simulink model "PIDforVerilog"  (R2024b)
settings: Solver=VariableStepAuto  StartTime=0.0  StopTime=10.0  RelTol=1e-3
undefined symbols (not defined in the file): DiscIntNeverNeededParam
libraries: simulink x6
(part 3 of 3)

== system PIDforVerilog/Discrete PID Controller/Filter/Passthrough ==
  Reset : Inport  SampleTime=SampleTime
  U : Inport  Port=2  SampleTime=SampleTime
  N : Inport  Port=3  SampleTime=SampleTime
  D0in : Inport  Port=4  SampleTime=SampleTime
  Nout : Inport  Port=5  SampleTime=SampleTime
  Ts : Inport  Port=6  SampleTime=SampleTime
  Signal Specification1 : SignalSpecification  DisableCoverage=on  OutDataTypeStr=boolean  SampleTime=SampleTime
  Signal Specification4 : SignalSpecification  DisableCoverage=on  OutDataTypeStr=boolean  SampleTime=SampleTime
  Terminator{1..2,4..6} (5 alike) : Terminator
  Y : Outport  SampleTime=SampleTime
  wires:
  Nout/1 -> Terminator2/1
  Reset/1 -> Terminator5/1
  D0in/1 -> Signal Specification4/1
  Signal Specification4/1 -> Terminator4/1
  N/1 -> Signal Specification1/1
  Signal Specification1/1 -> Terminator1/1
  U/1 -> Y/1
  Ts/1 -> Terminator6/1

== system PIDforVerilog/Discrete PID Controller/Filter ICs/Disabled ==
  D0 : Inport  SampleTime=SampleTime
  Ground : Ground  DisableCoverage=on
  Signal Specification : SignalSpecification  DisableCoverage=on  OutDataTypeStr=boolean  SampleTime=SampleTime
  Signal Specification1 : SignalSpecification  DisableCoverage=on  OutDataTypeStr=boolean  SampleTime=SampleTime
  Terminator : Terminator
  Out1 : Outport  SampleTime=SampleTime
  wires:
  D0/1 -> Signal Specification/1
  Signal Specification/1 -> Terminator/1
  Ground/1 -> Signal Specification1/1
  Signal Specification1/1 -> Out1/1

== system PIDforVerilog/Discrete PID Controller/Filter ICs/External IC ==
  D0 : Inport  SampleTime=SampleTime
  Out1 : Outport  SampleTime=SampleTime
  wires:
  D0/1 -> Out1/1

== system PIDforVerilog/Discrete PID Controller/Filter ICs/Internal IC - Differentiator ==
  D0 : Inport  SampleTime=SampleTime
  Ground : Ground  DisableCoverage=on
  Signal Specification : SignalSpecification  DisableCoverage=on  OutDataTypeStr=boolean  SampleTime=SampleTime
  Signal Specification1 : SignalSpecification  DisableCoverage=on  OutDataTypeStr=boolean  SampleTime=SampleTime
  Terminator : Terminator
  Out1 : Outport  SampleTime=SampleTime
  wires:
  D0/1 -> Signal Specification/1
  Signal Specification/1 -> Terminator/1
  Ground/1 -> Signal Specification1/1
  Signal Specification1/1 -> Out1/1

== system PIDforVerilog/Discrete PID Controller/Filter ICs/Internal IC - Filter ==
  D0 : Inport  OutDataTypeStr=fixdt(1,32,16, 'DataTypeOverride', 'Off')  PortDimensions=1  SampleTime=SampleTime
  Ground : Ground  DisableCoverage=on
  Terminator : Terminator
  Out1 : Outport  OutDataTypeStr=fixdt(1,32,16, 'DataTypeOverride', 'Off')  SampleTime=SampleTime
  wires:
  D0/1 -> Terminator/1
  Ground/1 -> Out1/1

== system PIDforVerilog/Discrete PID Controller/I Gain/Disabled ==
  I Gain : Inport  SampleTime=SampleTime
  Signal Specification : SignalSpecification  DisableCoverage=on  OutDataTypeStr=boolean  SampleTime=SampleTime
  Terminator : Terminator
  wires:
  Signal Specification/1 -> Terminator/1
  I Gain/1 -> Signal Specification/1

== system PIDforVerilog/Discrete PID Controller/I Gain/External Parameters ==
  err : Inport  SampleTime=SampleTime
  I Gain : Inport  Port=2  SampleTime=SampleTime
  IProd Out : Product  OutMin=IOutMin  OutMax=IOutMax  OutDataTypeStr=fixdt(1,32,16, 'DataTypeOverride', 'Off')  SaturateOnIntegerOverflow=on  SampleTime=SampleTime
  Out1 : Outport  SampleTime=SampleTime
  wires:
  err/1 -> IProd Out/1
  I Gain/1 -> IProd Out/2
  IProd Out/1 -> Out1/1

== system PIDforVerilog/Discrete PID Controller/I Gain/Internal Parameters ==
  err : Inport  SampleTime=SampleTime
  I Gain : Inport  Port=2  OutDataTypeStr=fixdt(1,32,16, 'DataTypeOverride', 'Off')  SampleTime=SampleTime
  Integral Gain : Gain  DisableCoverage=on  Gain=I  ParamMin=IParamMin  ParamMax=IParamMax  ParamDataTypeStr=fixdt(1,32,16, 'DataTypeOverride', 'Off')  OutMin=IOutMin  OutMax=IOutMax  OutDataTypeStr=fixdt(1,32,16, 'DataTypeOverride', 'Off')  SaturateOnIntegerOverflow=on
  Terminator : Terminator
  Out1 : Outport  OutDataTypeStr=fixdt(1,32,16, 'DataTypeOverride', 'Off')  SampleTime=SampleTime
  wires:
  err/1 -> Integral Gain/1
  Integral Gain/1 -> Out1/1
  I Gain/1 -> Terminator/1

== system PIDforVerilog/Discrete PID Controller/Ideal P Gain/External Parameters ==
  In1 : Inport  SampleTime=SampleTime
  P Gain : Inport  Port=2  SampleTime=SampleTime
  PProd Out : Product  OutDataTypeStr=fixdt(1,32,16, 'DataTypeOverride', 'Off')  SaturateOnIntegerOverflow=on  SampleTime=SampleTime
  Out1 : Outport  SampleTime=SampleTime
  wires:
  In1/1 -> PProd Out/1
  P Gain/1 -> PProd Out/2
  PProd Out/1 -> Out1/1

== system PIDforVerilog/Discrete PID Controller/Ideal P Gain/Internal Parameters ==
  In1 : Inport  SampleTime=SampleTime
  P Gain : Inport  Port=2  SampleTime=SampleTime
  Proportional Gain : Gain  Gain=P  ParamMin=PParamMin  ParamMax=PParamMax  ParamDataTypeStr=fixdt(1,32,16, 'DataTypeOverride', 'Off')  OutMin=POutMin  OutMax=POutMax  OutDataTypeStr=fixdt(1,32,16, 'DataTypeOverride', 'Off')  SaturateOnIntegerOverflow=on
  Signal Specification1 : SignalSpecification  DisableCoverage=on  OutDataTypeStr=boolean  SampleTime=SampleTime
  Terminator1 : Terminator
  Out1 : Outport  SampleTime=SampleTime
  wires:
  In1/1 -> Proportional Gain/1
  Proportional Gain/1 -> Out1/1
  P Gain/1 -> Signal Specification1/1
  Signal Specification1/1 -> Terminator1/1

== system PIDforVerilog/Discrete PID Controller/Ideal P Gain/Passthrough ==
  In1 : Inport  SampleTime=SampleTime
  P Gain : Inport  Port=2  SampleTime=SampleTime
  Terminator1 : Terminator
  Out1 : Outport  SampleTime=SampleTime
  wires:
  In1/1 -> Out1/1
  P Gain/1 -> Terminator1/1

== system PIDforVerilog/Discrete PID Controller/Ideal P Gain Fdbk/Disabled ==
  In1 : Inport  OutDataTypeStr=fixdt(1,32,16, 'DataTypeOverride', 'Off')  SampleTime=SampleTime
  P Gain : Inport  Port=2  SampleTime=SampleTime
  Terminator1 : Terminator
  Terminator2 : Terminator
  wires:
  P Gain/1 -> Terminator1/1
  In1/1 -> Terminator2/1

== system PIDforVerilog/Discrete PID Controller/Ideal P Gain Fdbk/External Parameters ==
  In1 : Inport  SampleTime=SampleTime
  P Gain : Inport  Port=2  SampleTime=SampleTime
  PProd Out : Product  OutDataTypeStr=fixdt(1,32,16, 'DataTypeOverride', 'Off')  SaturateOnIntegerOverflow=on  SampleTime=SampleTime
  Out1 : Outport  SampleTime=SampleTime
  wires:
  PProd Out/1 -> Out1/1
  P Gain/1 -> PProd Out/2
  In1/1 -> PProd Out/1

== system PIDforVerilog/Discrete PID Controller/Ideal P Gain Fdbk/Internal Parameters ==
  In1 : Inport  SampleTime=SampleTime
  P Gain : Inport  Port=2  SampleTime=SampleTime
  Proportional Gain : Gain  Gain=P  ParamMin=PParamMin  ParamMax=PParamMax  ParamDataTypeStr=fixdt(1,32,16, 'DataTypeOverride', 'Off')  OutMin=POutMin  OutMax=POutMax  OutDataTypeStr=fixdt(1,32,16, 'DataTypeOverride', 'Off')  SaturateOnIntegerOverflow=on
  Signal Specification1 : SignalSpecification  DisableCoverage=on  OutDataTypeStr=boolean  SampleTime=SampleTime
  Terminator1 : Terminator
  Out1 : Outport  SampleTime=SampleTime
  wires:
  Proportional Gain/1 -> Out1/1
  In1/1 -> Proportional Gain/1
  Signal Specification1/1 -> Terminator1/1
  P Gain/1 -> Signal Specification1/1

== system PIDforVerilog/Discrete PID Controller/Ideal P Gain Fdbk/Passthrough ==
  In1 : Inport  SampleTime=SampleTime
  P Gain : Inport  Port=2  SampleTime=SampleTime
  Terminator1 : Terminator
  Out1 : Outport  SampleTime=SampleTime
  wires:
  In1/1 -> Out1/1
  P Gain/1 -> Terminator1/1

== system PIDforVerilog/Discrete PID Controller/Integrator/Continuous ==
  U : Inport  SampleTime=SampleTime
  Reset : Inport  Port=2  SampleTime=SampleTime
  I0in : Inport  Port=3  SampleTime=SampleTime
  Ground : Ground  DisableCoverage=on
  Integrator : Integrator  InitialCondition=InitialConditionForIntegrator  LimitOutput=on  UpperSaturationLimit=UpperIntegratorSaturationLimit  LowerSaturationLimit=LowerIntegratorSaturationLimit  ZeroCross=off
  Signal Specification1 : SignalSpecification  DisableCoverage=on  OutDataTypeStr=boolean  SampleTime=SampleTime
  Terminator : Terminator
  Terminator1 : Terminator
  state : Outport  SampleTime=SampleTime
  out : Outport  Port=2  SampleTime=SampleTime
  wires:
  U/1 -> Integrator/1
  I0in/1 -> Terminator/1
  Integrator/1 -> out/1
  Ground/1 -> Signal Specification1/1
  Signal Specification1/1 -> state/1
  Reset/1 -> Terminator1/1

== system PIDforVerilog/Discrete PID Controller/Integrator/Disabled ==
  U : Inport  SampleTime=SampleTime
  Reset : Inport  Port=2  SampleTime=SampleTime
  I0in : Inport  Port=3  SampleTime=SampleTime
  Ground : Ground  DisableCoverage=on
  Signal Specification1 : SignalSpecification  DisableCoverage=on  OutDataTypeStr=boolean  SampleTime=SampleTime
  Signal Specification2 : SignalSpecification  DisableCoverage=on  OutDataTypeStr=boolean  SampleTime=SampleTime
  Signal Specification4 : SignalSpecification  DisableCoverage=on  OutDataTypeStr=boolean  SampleTime=SampleTime
  Terminator1 : Terminator
  Terminator2 : Terminator
  Terminator3 : Terminator
  out : Outport  SampleTime=SampleTime
  wires:
  Reset/1 -> Terminator2/1
  Signal Specification4/1 -> Terminator1/1
  I0in/1 -> Signal Specification4/1
  U/1 -> Signal Specification1/1
  Signal Specification1/1 -> Terminator3/1
  Ground/1 -> Signal Specification2/1
  Signal Specification2/1 -> out/1

== system PIDforVerilog/Discrete PID Controller/Integrator/Discrete ==
  U : Inport  SampleTime=SampleTime
  Reset : Inport  Port=2  SampleTime=SampleTime
  I0in : Inport  Port=3  SampleTime=SampleTime
  Ground_Integrator : Ground  DisableCoverage=on
  Integrator : DiscreteIntegrator  InitialCondition=InitialConditionForIntegrator  SampleTime=SampleTime  OutMin=IntegratorOutMin  OutMax=IntegratorOutMax  OutDataTypeStr=fixdt(1,32,16, 'DataTypeOverride', 'Off')  SaturateOnIntegerOverflow=on  LimitOutput=on  UpperSaturationLimit=UpperIntegratorSaturationLimit  LowerSaturationLimit=LowerIntegratorSaturationLimit  ICPrevOutput=DiscIntNeverNeededParam  ICPrevScaledInput=DiscIntNeverNeededParam
  Terminator : Terminator
  Terminator1 : Terminator
  Terminator2 : Terminator
  out : Outport  SampleTime=SampleTime
  state : Outport  Port=2  SampleTime=SampleTime
  wires:
  I0in/1 -> Terminator1/1
  Integrator/1 -> out/1
  U/1 -> Integrator/1
  Ground_Integrator/1 -> Terminator/1, state/1
  Reset/1 -> Terminator2/1

== system PIDforVerilog/Discrete PID Controller/Integrator ICs/Disabled ==
  I0 : Inport  SampleTime=SampleTime
  Ground : Ground  DisableCoverage=on
  Signal Specification : SignalSpecification  DisableCoverage=on  OutDataTypeStr=boolean  SampleTime=SampleTime
  Signal Specification1 : SignalSpecification  DisableCoverage=on  OutDataTypeStr=boolean  SampleTime=SampleTime
  Terminator : Terminator
  Out1 : Outport  SampleTime=SampleTime
  wires:
  Signal Specification/1 -> Terminator/1
  I0/1 -> Signal Specification/1
  Signal Specification1/1 -> Out1/1
  Ground/1 -> Signal Specification1/1

== system PIDforVerilog/Discrete PID Controller/Integrator ICs/External IC ==
  I0 : Inport  SampleTime=SampleTime
  Out1 : Outport  SampleTime=SampleTime
  wires:
  I0/1 -> Out1/1

== system PIDforVerilog/Discrete PID Controller/Integrator ICs/Internal IC ==
  I0 : Inport  OutDataTypeStr=fixdt(1,32,16, 'DataTypeOverride', 'Off')  SampleTime=SampleTime
  Ground : Ground  DisableCoverage=on
  Terminator : Terminator
  Out1 : Outport  OutDataTypeStr=fixdt(1,32,16, 'DataTypeOverride', 'Off')  SampleTime=SampleTime
  wires:
  I0/1 -> Terminator/1
  Ground/1 -> Out1/1

== system PIDforVerilog/Discrete PID Controller/N Copy/Disabled ==
  N Gain : Inport  OutDataTypeStr=fixdt(1,32,16, 'DataTypeOverride', 'Off')  SampleTime=SampleTime
  Terminator : Terminator
  wires:
  N Gain/1 -> Terminator/1

== system PIDforVerilog/Discrete PID Controller/N Copy/Disabled wSignal Specification ==
  N Gain : Inport  SampleTime=SampleTime
  Signal Specification1 : SignalSpecification  DisableCoverage=on  OutDataTypeStr=boolean  SampleTime=SampleTime
  Terminator : Terminator
  wires:
  N Gain/1 -> Signal Specification1/1
  Signal Specification1/1 -> Terminator/1

== system PIDforVerilog/Discrete PID Controller/N Copy/External Parameters ==
  N Gain : Inport  SampleTime=SampleTime
  Out1 : Outport  SampleTime=SampleTime
  wires:
  N Gain/1 -> Out1/1

== system PIDforVerilog/Discrete PID Controller/N Copy/Internal Parameters ==
  N Gain : Inport  SampleTime=SampleTime
  N Copy : Constant  DisableCoverage=on  Value=N  OutMin=NCopyOutMin  OutMax=NCopyOutMax  OutDataTypeStr=fixdt(1,32,16, 'DataTypeOverride', 'Off')  PreserveConstantTs=on
  Signal Specification : SignalSpecification  DisableCoverage=on  OutDataTypeStr=boolean  SampleTime=SampleTime
  Terminator : Terminator
  Out1 : Outport  SampleTime=SampleTime
  wires:
  N Copy/1 -> Out1/1
  N Gain/1 -> Signal Specification/1
  Signal Specification/1 -> Terminator/1

== system PIDforVerilog/Discrete PID Controller/N Gain/Disabled ==
  U : Inport  SampleTime=SampleTime
  N Gain : Inport  Port=2  SampleTime=SampleTime
  Signal Specification1 : SignalSpecification  DisableCoverage=on  OutDataTypeStr=boolean  SampleTime=SampleTime
  Signal Specification2 : SignalSpecification  DisableCoverage=on  OutDataTypeStr=boolean  SampleTime=SampleTime
  Terminator1 : Terminator
  Terminator2 : Terminator
  wires:
  Signal Specification2/1 -> Terminator2/1
  U/1 -> Signal Specification2/1
  N Gain/1 -> Signal Specification1/1
  Signal Specification1/1 -> Terminator1/1

== system PIDforVerilog/Discrete PID Controller/N Gain/External Parameters ==
  U : Inport  SampleTime=SampleTime
  N Gain : Inport  Port=2  SampleTime=SampleTime
  NProd Out : Product  OutMin=NOutMin  OutMax=NOutMax  OutDataTypeStr=fixdt(1,32,16, 'DataTypeOverride', 'Off')  SaturateOnIntegerOverflow=on  SampleTime=SampleTime
  Out1 : Outport  SampleTime=SampleTime
  wires:
  U/1 -> NProd Out/1
  N Gain/1 -> NProd Out/2
  NProd Out/1 -> Out1/1

== system PIDforVerilog/Discrete PID Controller/N Gain/Internal Parameters ==
  U : Inport  SampleTime=SampleTime
  N Gain : Inport  Port=2  SampleTime=SampleTime
  Filter Coefficient : Gain  Gain=N  ParamMin=NParamMin  ParamMax=NParamMax  ParamDataTypeStr=fixdt(1,32,16, 'DataTypeOverride', 'Off')  OutMin=NOutMin  OutMax=NOutMax  OutDataTypeStr=fixdt(1,32,16, 'DataTypeOverride', 'Off')  SaturateOnIntegerOverflow=on
  Terminator1 : Terminator
  Out1 : Outport  SampleTime=SampleTime
  wires:
  U/1 -> Filter Coefficient/1
  Filter Coefficient/1 -> Out1/1
  N Gain/1 -> Terminator1/1

== system PIDforVerilog/Discrete PID Controller/N Gain/Passthrough ==
  U : Inport  SampleTime=SampleTime
  N Gain : Inport  Port=2  SampleTime=SampleTime
  Terminator1 : Terminator
  Out1 : Outport  SampleTime=SampleTime
  wires:
  U/1 -> Out1/1
  N Gain/1 -> Terminator1/1

== system PIDforVerilog/Discrete PID Controller/P Copy/Disabled ==
  P Gain : Inport  SampleTime=SampleTime
  Terminator3 : Terminator
  wires:
  P Gain/1 -> Terminator3/1

== system PIDforVerilog/Discrete PID Controller/P Copy/External Parameters Ideal ==
  P Gain : Inport  SampleTime=SampleTime
  Out1 : Outport  SampleTime=SampleTime
  wires:
  P Gain/1 -> Out1/1

== system PIDforVerilog/Discrete PID Controller/P Copy/Internal Parameters Ideal ==
  P Gain : Inport  SampleTime=SampleTime
  P Copy : Constant  DisableCoverage=on  Value=P  OutMin=PCopyOutMin  OutMax=PCopyOutMax  OutDataTypeStr=Inherit: Inherit via back propagation  PreserveConstantTs=on
  Terminator3 : Terminator
  Out1 : Outport  SampleTime=SampleTime
  wires:
  P Copy/1 -> Out1/1
  P Gain/1 -> Terminator3/1

== system PIDforVerilog/Discrete PID Controller/Parallel P Gain/Disabled ==
  P Gain : Inport  SampleTime=SampleTime
  Signal Specification : SignalSpecification  DisableCoverage=on  OutDataTypeStr=boolean  SampleTime=SampleTime
  Terminator : Terminator
  wires:
  P Gain/1 -> Signal Specification/1
  Signal Specification/1 -> Terminator/1

== system PIDforVerilog/Discrete PID Controller/Parallel P Gain/External Parameters ==
  err : Inport  SampleTime=SampleTime
  P Gain : Inport  Port=2  SampleTime=SampleTime
  PProd Out : Product  OutMin=POutMin  OutMax=POutMax  OutDataTypeStr=fixdt(1,32,16, 'DataTypeOverride', 'Off')  SaturateOnIntegerOverflow=on  SampleTime=SampleTime
  Out1 : Outport  SampleTime=SampleTime
  wires:
  PProd Out/1 -> Out1/1
  P Gain/1 -> PProd Out/2
  err/1 -> PProd Out/1

== system PIDforVerilog/Discrete PID Controller/Parallel P Gain/Internal Parameters ==
  err : Inport  SampleTime=SampleTime
  P Gain : Inport  Port=2  OutDataTypeStr=fixdt(1,32,16, 'DataTypeOverride', 'Off')  SampleTime=SampleTime
  Proportional Gain : Gain  Gain=P  ParamMin=PParamMin  ParamMax=PParamMax  ParamDataTypeStr=fixdt(1,32,16, 'DataTypeOverride', 'Off')  OutMin=POutMin  OutMax=POutMax  OutDataTypeStr=fixdt(1,32,16, 'DataTypeOverride', 'Off')  SaturateOnIntegerOverflow=on
  Terminator : Terminator
  Out1 : Outport  SampleTime=SampleTime
  wires:
  Proportional Gain/1 -> Out1/1
  err/1 -> Proportional Gain/1
  P Gain/1 -> Terminator/1

== system PIDforVerilog/Discrete PID Controller/Parallel P Gain/Passthrough ==
  err : Inport  SampleTime=SampleTime
  P Gain : Inport  Port=2  SampleTime=SampleTime
  Terminator : Terminator
  Out1 : Outport  SampleTime=SampleTime
  wires:
  err/1 -> Out1/1
  P Gain/1 -> Terminator/1

== system PIDforVerilog/Discrete PID Controller/Reset Signal/Disabled ==
  Reset : Inport  OutDataTypeStr=fixdt(1,32,16, 'DataTypeOverride', 'Off')  SampleTime=SampleTime
  Ground : Ground  DisableCoverage=on
  Terminator : Terminator
  Out1 : Outport  OutDataTypeStr=fixdt(1,32,16, 'DataTypeOverride', 'Off')  SampleTime=SampleTime
  wires:
  Reset/1 -> Terminator/1
  Ground/1 -> Out1/1

== system PIDforVerilog/Discrete PID Controller/Reset Signal/External Reset ==
  Reset : Inport  SampleTime=SampleTime
  Out1 : Outport  SampleTime=SampleTime
  wires:
  Reset/1 -> Out1/1

== system PIDforVerilog/Discrete PID Controller/Saturation/Enabled ==
  In1 : Inport  SampleTime=SampleTime
  Upper Limit : Inport  Port=2  OutDataTypeStr=fixdt(1,32,16, 'DataTypeOverride', 'Off')  SampleTime=SampleTime
  Lower Limit : Inport  Port=3  OutDataTypeStr=fixdt(1,32,16, 'DataTypeOverride', 'Off')  SampleTime=SampleTime
  Saturation : Saturate  UpperLimit=UpperSaturationLimit  LowerLimit=LowerSaturationLimit  ZeroCross=off  SampleTime=SampleTime  OutMin=SaturationOutMin  OutMax=SaturationOutMax  OutDataTypeStr=fixdt(1,32,16, 'DataTypeOverride', 'Off')
  Terminator : Terminator
  Terminator1 : Terminator
  Out1 : Outport  SampleTime=SampleTime
  wires:
  Lower Limit/1 -> Terminator1/1
  Upper Limit/1 -> Terminator/1
  In1/1 -> Saturation/1
  Saturation/1 -> Out1/1

== system PIDforVerilog/Discrete PID Controller/Saturation/External ==
  In1 : Inport  SampleTime=SampleTime
  Upper Limit : Inport  Port=2  SampleTime=SampleTime
  Lower Limit : Inport  Port=3  SampleTime=SampleTime
  Saturation Dynamic : simulink/Discontinuities/Saturation Dynamic  OutMin=SaturationOutMin  OutMax=SaturationOutMax  OutDataTypeStr=Inherit: Same as second input  OutDataType=fixdt(1, 16)  OutScaling=2^-10  DoSatur=on
  Out1 : Outport  SampleTime=SampleTime
  wires:
  Lower Limit/1 -> Saturation Dynamic/3
  Upper Limit/1 -> Saturation Dynamic/1
  Saturation Dynamic/1 -> Out1/1
  In1/1 -> Saturation Dynamic/2

== system PIDforVerilog/Discrete PID Controller/Saturation/Passthrough ==
  In1 : Inport  SampleTime=SampleTime
  Upper Limit : Inport  Port=2  SampleTime=SampleTime
  Lower Limit : Inport  Port=3  SampleTime=SampleTime
  Signal Specification : SignalSpecification  DisableCoverage=on  OutDataTypeStr=boolean  SampleTime=SampleTime
  Signal Specification1 : SignalSpecification  DisableCoverage=on  OutDataTypeStr=boolean  SampleTime=SampleTime
  Terminator : Terminator
  Terminator1 : Terminator
  Out1 : Outport  SampleTime=SampleTime
  wires:
  Signal Specification1/1 -> Terminator1/1
  Lower Limit/1 -> Signal Specification1/1
  Upper Limit/1 -> Signal Specification/1
  Signal Specification/1 -> Terminator/1
  In1/1 -> Out1/1

== system PIDforVerilog/Discrete PID Controller/Saturation Fdbk/Disabled ==
  In1 : Inport  OutDataTypeStr=fixdt(1,32,16, 'DataTypeOverride', 'Off')  SampleTime=SampleTime
  Terminator1 : Terminator
  wires:
  In1/1 -> Terminator1/1

== system PIDforVerilog/Discrete PID Controller/Saturation Fdbk/Enabled ==
  In1 : Inport  SampleTime=SampleTime
  Saturation : Saturate  UpperLimit=UpperSaturationLimit  LowerLimit=LowerSaturationLimit  ZeroCross=off  SampleTime=SampleTime  OutMin=SaturationOutMin  OutMax=SaturationOutMax  OutDataTypeStr=fixdt(1,32,16, 'DataTypeOverride', 'Off')
  Out1 : Outport  SampleTime=SampleTime
  wires:
  Saturation/1 -> Out1/1
  In1/1 -> Saturation/1

== system PIDforVerilog/Discrete PID Controller/Saturation Fdbk/External ==
  In1 : Inport  SampleTime=SampleTime
  Upper Limit : Inport  Port=2  SampleTime=SampleTime
  Lower Limit : Inport  Port=3  SampleTime=SampleTime
  Saturation Dynamic : simulink/Discontinuities/Saturation Dynamic  OutMin=SaturationOutMin  OutMax=SaturationOutMax  OutDataTypeStr=Inherit: Same as second input  OutDataType=fixdt(1, 16)  OutScaling=2^-10  DoSatur=on
  Out1 : Outport  SampleTime=SampleTime
  wires:
  Lower Limit/1 -> Saturation Dynamic/3
  Upper Limit/1 -> Saturation Dynamic/1
  Saturation Dynamic/1 -> Out1/1
  In1/1 -> Saturation Dynamic/2

== system PIDforVerilog/Discrete PID Controller/Saturation Fdbk/Passthrough ==
  In1 : Inport  SampleTime=SampleTime
  Out1 : Outport  SampleTime=SampleTime
  wires:
  In1/1 -> Out1/1

== system PIDforVerilog/Discrete PID Controller/Sum/Passthrough_I ==
  P : Inport  SampleTime=SampleTime
  I : Inport  Port=2  SampleTime=SampleTime
  Signal Specification : SignalSpecification  OutDataTypeStr=boolean  SampleTime=SampleTime
  Terminator : Terminator
  Out1 : Outport  SampleTime=SampleTime
  wires:
  Signal Specification/1 -> Terminator/1
  P/1 -> Signal Specification/1
  I/1 -> Out1/1

== system PIDforVerilog/Discrete PID Controller/Sum/Passthrough_P ==
  P : Inport  SampleTime=SampleTime
  Out1 : Outport  SampleTime=SampleTime
  wires:
  P/1 -> Out1/1

== system PIDforVerilog/Discrete PID Controller/Sum/Sum_PD ==
  P : Inport  SampleTime=SampleTime
  D : Inport  Port=2  SampleTime=SampleTime
  Sum : Sum  Inputs=|++  OutMin=SumOutMin  OutMax=SumOutMax  OutDataTypeStr=fixdt(1,32,16, 'DataTypeOverride', 'Off')  AccumDataTypeStr=fixdt(1,32,16, 'DataTypeOverride', 'Off')  SaturateOnIntegerOverflow=on
  Out1 : Outport  SampleTime=SampleTime
  wires:
  P/1 -> Sum/1
  D/1 -> Sum/2
  Sum/1 -> Out1/1

== system PIDforVerilog/Discrete PID Controller/Sum/Sum_PI ==
  P : Inport  SampleTime=SampleTime
  I : Inport  Port=2  SampleTime=SampleTime
  Sum : Sum  Inputs=|++  OutMin=SumOutMin  OutMax=SumOutMax  OutDataTypeStr=fixdt(1,32,16, 'DataTypeOverride', 'Off')  AccumDataTypeStr=fixdt(1,32,16, 'DataTypeOverride', 'Off')  SaturateOnIntegerOverflow=on
  Out1 : Outport  SampleTime=SampleTime
  wires:
  I/1 -> Sum/2
  P/1 -> Sum/1
  Sum/1 -> Out1/1

== system PIDforVerilog/Discrete PID Controller/Sum/Sum_PID ==
  P : Inport  SampleTime=SampleTime
  I : Inport  Port=2  SampleTime=SampleTime
  D : Inport  Port=3  SampleTime=SampleTime
  Sum : Sum  Inputs=+++  OutMin=SumOutMin  OutMax=SumOutMax  OutDataTypeStr=fixdt(1,32,16, 'DataTypeOverride', 'Off')  AccumDataTypeStr=fixdt(1,32,16, 'DataTypeOverride', 'Off')  SaturateOnIntegerOverflow=on
  Out1 : Outport  SampleTime=SampleTime
  wires:
  I/1 -> Sum/2
  P/1 -> Sum/1
  D/1 -> Sum/3
  Sum/1 -> Out1/1

== system PIDforVerilog/Discrete PID Controller/Sum Fdbk/Disabled ==
  fromP : Inport  SampleTime=SampleTime
  fromState : Inport  Port=2  OutDataTypeStr=fixdt(1,32,16, 'DataTypeOverride', 'Off')  SampleTime=SampleTime
  fromD : Inport  Port=3  SampleTime=SampleTime
  Terminator1 : Terminator
  Terminator2 : Terminator
  Terminator3 : Terminator
  wires:
  fromD/1 -> Terminator3/1
  fromP/1 -> Terminator1/1
  fromState/1 -> Terminator2/1

== system PIDforVerilog/Discrete PID Controller/Sum Fdbk/Enabled ==
  fromP : Inport  SampleTime=SampleTime
  fromState : Inport  Port=2  SampleTime=SampleTime
  fromD : Inport  Port=3  SampleTime=SampleTime
  Sum Fdbk : Sum  DisableCoverage=on  Inputs=+++  OutMin=SumOutMin  OutMax=SumOutMax  OutDataTypeStr=fixdt(1,32,16, 'DataTypeOverride', 'Off')  AccumDataTypeStr=fixdt(1,32,16, 'DataTypeOverride', 'Off')  SaturateOnIntegerOverflow=on
  Out1 : Outport  SampleTime=SampleTime
  wires:
  fromP/1 -> Sum Fdbk/1
  fromState/1 -> Sum Fdbk/2
  fromD/1 -> Sum Fdbk/3
  Sum Fdbk/1 -> Out1/1

== system PIDforVerilog/Discrete PID Controller/Sum Fdbk/Passthrough ==
  fromState : Inport  SampleTime=SampleTime
  Out1 : Outport  SampleTime=SampleTime
  wires:
  fromState/1 -> Out1/1

== system PIDforVerilog/Discrete PID Controller/Tracking Mode/Disabled ==
  uout : Inport  SampleTime=SampleTime
  TR : Inport  Port=2  OutDataTypeStr=fixdt(1,32,16, 'DataTypeOverride', 'Off')  SampleTime=SampleTime
  Terminator1 : Terminator
  Terminator3 : Terminator
  wires:
  uout/1 -> Terminator3/1
  TR/1 -> Terminator1/1

== system PIDforVerilog/Discrete PID Controller/Tracking Mode/Enabled ==
  uout : Inport  SampleTime=SampleTime
  TR : Inport  Port=2  SampleTime=SampleTime
  Kt : Gain  Gain=Kt  ParamMin=KtParamMin  ParamMax=KtParamMax  OutMin=KtOutMin  OutMax=KtOutMax  SaturateOnIntegerOverflow=on
  SumI3 : Sum  Inputs=|-+  OutMin=SumI3OutMin  OutMax=SumI3OutMax  SaturateOnIntegerOverflow=on
  Out1 : Outport  SampleTime=SampleTime
  wires:
  Kt/1 -> Out1/1
  SumI3/1 -> Kt/1
  TR/1 -> SumI3/2
  uout/1 -> SumI3/1

== system PIDforVerilog/Discrete PID Controller/Tracking Mode Sum/Passthrough ==
  fromIgain : Inport  SampleTime=SampleTime
  fromTR : Inport  Port=2  OutDataTypeStr=fixdt(1,32,16, 'DataTypeOverride', 'Off')  SampleTime=SampleTime
  Signal Specification : SignalSpecification  Commented=on  DisableCoverage=on  OutDataTypeStr=fixdt(0,1, 'DataTypeOverride', 'Off')  Dimensions=1  SampleTime=SampleTime
  Terminator : Terminator
  preInt : Outport
  wires:
  fromIgain/1 -> preInt/1
  fromTR/1 -> Terminator/1

== system PIDforVerilog/Discrete PID Controller/Tracking Mode Sum/Tracking Mode ==
  fromIgain : Inport  SampleTime=SampleTime
  fromTR : Inport  Port=2  SampleTime=SampleTime
  SumI1 : Sum  Inputs=|++  OutMin=SumI1OutMin  OutMax=SumI1OutMax  SaturateOnIntegerOverflow=on
  preInt : Outport
  wires:
  fromIgain/1 -> SumI1/1
  fromTR/1 -> SumI1/2
  SumI1/1 -> preInt/1

== system PIDforVerilog/Discrete PID Controller/Tsamp - Integral/Disabled ==
  U : Inport  SampleTime=SampleTime
  Ts : Inport  Port=2  SampleTime=SampleTime
  Terminator : Terminator
  Out1 : Outport  SampleTime=SampleTime
  wires:
  U/1 -> Out1/1
  Ts/1 -> Terminator/1

== system PIDforVerilog/Discrete PID Controller/Tsamp - Integral/External Ts ==
  U : Inport  SampleTime=SampleTime
  Ts : Inport  Port=2  SampleTime=SampleTime
  Uintegral*Ts Prod Out : Product  OutMin=UintegralTsProdOutMin  OutMax=UintegralTsProdOutMax  SaturateOnIntegerOverflow=on  SampleTime=SampleTime
  Out1 : Outport  SampleTime=SampleTime
  wires:
  U/1 -> Uintegral*Ts Prod Out/1
  Uintegral*Ts Prod Out/1 -> Out1/1
  Ts/1 -> Uintegral*Ts Prod Out/2

== system PIDforVerilog/Discrete PID Controller/Tsamp - Integral/Passthrough ==
  U : Inport  SampleTime=SampleTime
  Ts : Inport  Port=2  SampleTime=SampleTime
  Terminator : Terminator
  Out1 : Outport  SampleTime=SampleTime
  wires:
  Ts/1 -> Terminator/1
  U/1 -> Out1/1

== system PIDforVerilog/Discrete PID Controller/Tsamp - Integral/TsSignalSpecification ==
  U : Inport  SampleTime=SampleTime
  Ts : Inport  Port=2  OutDataTypeStr=fixdt(1,32,16, 'DataTypeOverride', 'Off')  SampleTime=SampleTime
  Terminator : Terminator
  Out1 : Outport  SampleTime=SampleTime
  wires:
  U/1 -> Out1/1
  Ts/1 -> Terminator/1

== system PIDforVerilog/Discrete PID Controller/Tsamp - Ngain/External Ts ==
  U : Inport  SampleTime=SampleTime
  Ts : Inport  Port=2  SampleTime=SampleTime
  Ungain*Ts Prod Out : Product  OutMin=UngainTsProdOutMin  OutMax=UngainTsProdOutMax  SaturateOnIntegerOverflow=on  SampleTime=SampleTime
  Out1 : Outport  SampleTime=SampleTime
  wires:
  Ts/1 -> Ungain*Ts Prod Out/2
  Ungain*Ts Prod Out/1 -> Out1/1
  U/1 -> Ungain*Ts Prod Out/1

== system PIDforVerilog/Discrete PID Controller/Tsamp - Ngain/Passthrough ==
  U : Inport  SampleTime=SampleTime
  Ts : Inport  Port=2  SampleTime=SampleTime
  Terminator : Terminator
  Out1 : Outport  SampleTime=SampleTime
  wires:
  U/1 -> Out1/1
  Ts/1 -> Terminator/1

== system PIDforVerilog/Discrete PID Controller/postSat Signal/Feedback_Path ==
  feedback : Inport  SampleTime=SampleTime
  forward : Inport  Port=2  SampleTime=SampleTime
  Terminator1 : Terminator
  Out1 : Outport  SampleTime=SampleTime
  wires:
  feedback/1 -> Out1/1
  forward/1 -> Terminator1/1

== system PIDforVerilog/Discrete PID Controller/postSat Signal/Forward_Path ==
  feedback : Inport  OutDataTypeStr=fixdt(1,32,16, 'DataTypeOverride', 'Off')  SampleTime=SampleTime
  forward : Inport  Port=2  SampleTime=SampleTime
  Terminator1 : Terminator
  Out1 : Outport  SampleTime=SampleTime
  wires:
  forward/1 -> Out1/1
  feedback/1 -> Terminator1/1

== system PIDforVerilog/Discrete PID Controller/preInt Signal/External PreInt ==
  preInt : Inport  SampleTime=SampleTime
  extAW : Inport  Port=2  SampleTime=SampleTime
  Terminator1 : Terminator
  Out1 : Outport  SampleTime=SampleTime
  wires:
  preInt/1 -> Terminator1/1
  extAW/1 -> Out1/1

== system PIDforVerilog/Discrete PID Controller/preInt Signal/Internal PreInt ==
  preInt : Inport  SampleTime=SampleTime
  extAW : Inport  Port=2  OutDataTypeStr=fixdt(1,32,16, 'DataTypeOverride', 'Off')  SampleTime=SampleTime
  Terminator1 : Terminator
  Out1 : Outport  SampleTime=SampleTime
  wires:
  extAW/1 -> Terminator1/1
  preInt/1 -> Out1/1

== system PIDforVerilog/Discrete PID Controller/preSat Signal/Feedback_Path ==
  feedback : Inport  SampleTime=SampleTime
  forward : Inport  Port=2  SampleTime=SampleTime
  Terminator1 : Terminator
  Out1 : Outport  SampleTime=SampleTime
  wires:
  feedback/1 -> Out1/1
  forward/1 -> Terminator1/1

== system PIDforVerilog/Discrete PID Controller/preSat Signal/Forward_Path ==
  feedback : Inport  SampleTime=SampleTime
  forward : Inport  Port=2  SampleTime=SampleTime
  Terminator1 : Terminator
  Out1 : Outport  SampleTime=SampleTime
  wires:
  forward/1 -> Out1/1
  feedback/1 -> Terminator1/1

== system PIDforVerilog/Discrete PID Controller/Anti-windup/Cont. Clamping Ideal/Dead Zone ==
  preSat : Inport
  Upper Limit : Inport  Port=2  SampleTime=SampleTime
  Lower Limit : Inport  Port=3  SampleTime=SampleTime
  Disabled : Subsystem  VariantControl=Disabled
  Enabled : Subsystem  VariantControl=Enabled
  External : Subsystem  VariantControl=External
  DZ out : Outport

== system PIDforVerilog/Discrete PID Controller/Anti-windup/Cont. Clamping Parallel/Dead Zone ==
  preSat : Inport
  Upper Limit : Inport  Port=2  SampleTime=SampleTime
  Lower Limit : Inport  Port=3  SampleTime=SampleTime
  Disabled : Subsystem  VariantControl=Disabled
  Enabled : Subsystem  VariantControl=Enabled
  External : Subsystem  VariantControl=External
  DZ out : Outport

== system PIDforVerilog/Discrete PID Controller/Anti-windup/Disc. Clamping Ideal/Dead Zone ==
  preSat : Inport
  Upper Limit : Inport  Port=2  SampleTime=SampleTime
  Lower Limit : Inport  Port=3  SampleTime=SampleTime
  Disabled : Subsystem  VariantControl=Disabled
  Enabled : Subsystem  VariantControl=Enabled
  External : Subsystem  VariantControl=External
  DZ out : Outport

== system PIDforVerilog/Discrete PID Controller/Anti-windup/Disc. Clamping Parallel/Dead Zone ==
  preSat : Inport
  Upper Limit : Inport  Port=2  SampleTime=SampleTime
  Lower Limit : Inport  Port=3  SampleTime=SampleTime
  Disabled : Subsystem  VariantControl=Disabled
  Enabled : Subsystem  VariantControl=Enabled
  External : Subsystem  VariantControl=External
  DZ out : Outport

== system PIDforVerilog/Discrete PID Controller/Filter/Differentiator/Tsamp ==
  U : Inport  SampleTime=SampleTime
  Ts : Inport  Port=2  SampleTime=SampleTime
  External Ts : Subsystem  VariantControl=ExternalTs
  Internal Ts : Subsystem  VariantControl=InternalTs
  Out1 : Outport  SampleTime=SampleTime

== system PIDforVerilog/Discrete PID Controller/Filter/Disc. Backward Euler Filter/Tsamp ==
  N : Inport  SampleTime=SampleTime
  Ts : Inport  Port=2  SampleTime=SampleTime
  External Ts : Subsystem  VariantControl=ExternalTs
  Internal Ts : Subsystem  VariantControl=InternalTs
  Out1 : Outport  SampleTime=SampleTime

== system PIDforVerilog/Discrete PID Controller/Filter/Disc. Backward Euler Filter Only/Tsamp ==
  N : Inport  SampleTime=SampleTime
  Ts : Inport  Port=2  SampleTime=SampleTime
  External Ts : Subsystem  VariantControl=ExternalTs
  Internal Ts : Subsystem  VariantControl=InternalTs
  Out1 : Outport  SampleTime=SampleTime

== system PIDforVerilog/Discrete PID Controller/Filter/Disc. Trapezoidal Filter/Tsamp ==
  N : Inport  SampleTime=SampleTime
  Ts : Inport  Port=2  SampleTime=SampleTime
  External Ts : Subsystem  VariantControl=ExternalTs
  Internal Ts : Subsystem  VariantControl=InternalTs
  Out1 : Outport  SampleTime=SampleTime

== system PIDforVerilog/Discrete PID Controller/Filter/Disc. Trapezoidal Filter Only/Tsamp ==
  N : Inport  SampleTime=SampleTime
  Ts : Inport  Port=2  SampleTime=SampleTime
  External Ts : Subsystem  VariantControl=ExternalTs
  Internal Ts : Subsystem  VariantControl=InternalTs
  Out1 : Outport  SampleTime=SampleTime

== system PIDforVerilog/Discrete PID Controller/Anti-windup/Cont. Clamping Ideal/Dead Zone/Disabled ==

== system PIDforVerilog/Discrete PID Controller/Anti-windup/Cont. Clamping Ideal/Dead Zone/Enabled ==
  preSat : Inport
  DeadZone : DeadZone  DisableCoverage=on  LowerValue=LowerSaturationLimit  UpperValue=UpperSaturationLimit  ZeroCross=off
  DZ out : Outport
  wires:
  preSat/1 -> DeadZone/1
  DeadZone/1 -> DZ out/1

== system PIDforVerilog/Discrete PID Controller/Anti-windup/Cont. Clamping Ideal/Dead Zone/External ==
  preSat : Inport
  Upper Limit : Inport  Port=2  SampleTime=SampleTime
  Lower Limit : Inport  Port=3  SampleTime=SampleTime
  Dead Zone Dynamic : simulink/Discontinuities/Dead Zone Dynamic
  DZ out : Outport
  wires:
  preSat/1 -> Dead Zone Dynamic/2
  Lower Limit/1 -> Dead Zone Dynamic/3
  Upper Limit/1 -> Dead Zone Dynamic/1
  Dead Zone Dynamic/1 -> DZ out/1

== system PIDforVerilog/Discrete PID Controller/Anti-windup/Cont. Clamping Parallel/Dead Zone/Disabled ==

== system PIDforVerilog/Discrete PID Controller/Anti-windup/Cont. Clamping Parallel/Dead Zone/Enabled ==
  preSat : Inport
  DeadZone : DeadZone  DisableCoverage=on  LowerValue=LowerSaturationLimit  UpperValue=UpperSaturationLimit  ZeroCross=off
  DZ out : Outport
  wires:
  preSat/1 -> DeadZone/1
  DeadZone/1 -> DZ out/1

== system PIDforVerilog/Discrete PID Controller/Anti-windup/Cont. Clamping Parallel/Dead Zone/External ==
  preSat : Inport
  Upper Limit : Inport  Port=2  SampleTime=SampleTime
  Lower Limit : Inport  Port=3  SampleTime=SampleTime
  Dead Zone Dynamic : simulink/Discontinuities/Dead Zone Dynamic
  DZ out : Outport
  wires:
  preSat/1 -> Dead Zone Dynamic/2
  Lower Limit/1 -> Dead Zone Dynamic/3
  Upper Limit/1 -> Dead Zone Dynamic/1
  Dead Zone Dynamic/1 -> DZ out/1

== system PIDforVerilog/Discrete PID Controller/Anti-windup/Disc. Clamping Ideal/Dead Zone/Disabled ==

== system PIDforVerilog/Discrete PID Controller/Anti-windup/Disc. Clamping Ideal/Dead Zone/Enabled ==
  preSat : Inport
  DeadZone : DeadZone  DisableCoverage=on  LowerValue=LowerSaturationLimit  UpperValue=UpperSaturationLimit  ZeroCross=off
  DZ out : Outport
  wires:
  DeadZone/1 -> DZ out/1
  preSat/1 -> DeadZone/1

== system PIDforVerilog/Discrete PID Controller/Anti-windup/Disc. Clamping Ideal/Dead Zone/External ==
  preSat : Inport
  Upper Limit : Inport  Port=2  SampleTime=SampleTime
  Lower Limit : Inport  Port=3  SampleTime=SampleTime
  Dead Zone Dynamic : simulink/Discontinuities/Dead Zone Dynamic
  DZ out : Outport
  wires:
  Dead Zone Dynamic/1 -> DZ out/1
  Upper Limit/1 -> Dead Zone Dynamic/1
  Lower Limit/1 -> Dead Zone Dynamic/3
  preSat/1 -> Dead Zone Dynamic/2

== system PIDforVerilog/Discrete PID Controller/Anti-windup/Disc. Clamping Parallel/Dead Zone/Disabled ==

== system PIDforVerilog/Discrete PID Controller/Anti-windup/Disc. Clamping Parallel/Dead Zone/Enabled ==
  preSat : Inport
  DeadZone : DeadZone  DisableCoverage=on  LowerValue=LowerSaturationLimit  UpperValue=UpperSaturationLimit  ZeroCross=off
  DZ out : Outport
  wires:
  DeadZone/1 -> DZ out/1
  preSat/1 -> DeadZone/1

== system PIDforVerilog/Discrete PID Controller/Anti-windup/Disc. Clamping Parallel/Dead Zone/External ==
  preSat : Inport
  Upper Limit : Inport  Port=2  SampleTime=SampleTime
  Lower Limit : Inport  Port=3  SampleTime=SampleTime
  Dead Zone Dynamic : simulink/Discontinuities/Dead Zone Dynamic
  DZ out : Outport
  wires:
  Dead Zone Dynamic/1 -> DZ out/1
  Upper Limit/1 -> Dead Zone Dynamic/1
  Lower Limit/1 -> Dead Zone Dynamic/3
  preSat/1 -> Dead Zone Dynamic/2

== system PIDforVerilog/Discrete PID Controller/Filter/Differentiator/Tsamp/External Ts ==
  U : Inport  SampleTime=SampleTime
  Ts : Inport  Port=2  SampleTime=SampleTime
  Udiff*Ts Prod Out : Product  Inputs=*/  OutMin=UdiffTsProdOutMin  OutMax=UdiffTsProdOutMax  SaturateOnIntegerOverflow=on  SampleTime=SampleTime
  Out1 : Outport  SampleTime=SampleTime
  wires:
  U/1 -> Udiff*Ts Prod Out/1
  Udiff*Ts Prod Out/1 -> Out1/1
  Ts/1 -> Udiff*Ts Prod Out/2

== system PIDforVerilog/Discrete PID Controller/Filter/Differentiator/Tsamp/Internal Ts ==
  U : Inport  SampleTime=SampleTime
  Ts : Inport  Port=2  SampleTime=SampleTime
  Terminator : Terminator
  Tsamp : SampleTimeMath  TsampMathOp=/  TsampMathImp=Offline Scaling Adjustment  SaturateOnIntegerOverflow=on
  Out1 : Outport  SampleTime=SampleTime
  wires:
  U/1 -> Tsamp/1
  Ts/1 -> Terminator/1
  Tsamp/1 -> Out1/1

== system PIDforVerilog/Discrete PID Controller/Filter/Disc. Backward Euler Filter/Tsamp/External Ts ==
  N : Inport  SampleTime=SampleTime
  Ts : Inport  Port=2  SampleTime=SampleTime
  N*Ts Prod Out : Product  OutMin=NTsProdOutMin  OutMax=NTsProdOutMax  SaturateOnIntegerOverflow=on  SampleTime=SampleTime
  Out1 : Outport  SampleTime=SampleTime
  wires:
  Ts/1 -> N*Ts Prod Out/2
  N*Ts Prod Out/1 -> Out1/1
  N/1 -> N*Ts Prod Out/1

== system PIDforVerilog/Discrete PID Controller/Filter/Disc. Backward Euler Filter/Tsamp/Internal Ts ==
  N : Inport  SampleTime=SampleTime
  Ts : Inport  Port=2  SampleTime=SampleTime
  Terminator : Terminator
  Tsamp : SampleTimeMath  TsampMathOp=*  SaturateOnIntegerOverflow=on
  Out1 : Outport  SampleTime=SampleTime
  wires:
  Tsamp/1 -> Out1/1
  Ts/1 -> Terminator/1
  N/1 -> Tsamp/1

== system PIDforVerilog/Discrete PID Controller/Filter/Disc. Backward Euler Filter Only/Tsamp/External Ts ==
  N : Inport  SampleTime=SampleTime
  Ts : Inport  Port=2  SampleTime=SampleTime
  N*Ts Prod Out : Product  OutMin=NTsProdOutMin  OutMax=NTsProdOutMax  SampleTime=SampleTime
  Out1 : Outport  SampleTime=SampleTime
  wires:
  N/1 -> N*Ts Prod Out/1
  N*Ts Prod Out/1 -> Out1/1
  Ts/1 -> N*Ts Prod Out/2

== system PIDforVerilog/Discrete PID Controller/Filter/Disc. Backward Euler Filter Only/Tsamp/Internal Ts ==
  N : Inport  SampleTime=SampleTime
  Ts : Inport  Port=2  SampleTime=SampleTime
  Terminator : Terminator
  Tsamp : SampleTimeMath  TsampMathOp=*
  Out1 : Outport  SampleTime=SampleTime
  wires:
  N/1 -> Tsamp/1
  Ts/1 -> Terminator/1
  Tsamp/1 -> Out1/1

== system PIDforVerilog/Discrete PID Controller/Filter/Disc. Trapezoidal Filter/Tsamp/External Ts ==
  N : Inport  SampleTime=SampleTime
  Ts : Inport  Port=2  SampleTime=SampleTime
  Gain : Gain  Gain=0.5  SaturateOnIntegerOverflow=on
  N*Ts Prod Out : Product  OutMin=NTsProdOutMin  OutMax=NTsProdOutMax  SaturateOnIntegerOverflow=on  SampleTime=SampleTime
  Out1 : Outport  SampleTime=SampleTime
  wires:
  Gain/1 -> N*Ts Prod Out/2
  Ts/1 -> Gain/1
  N*Ts Prod Out/1 -> Out1/1
  N/1 -> N*Ts Prod Out/1

== system PIDforVerilog/Discrete PID Controller/Filter/Disc. Trapezoidal Filter/Tsamp/Internal Ts ==
  N : Inport  SampleTime=SampleTime
  Ts : Inport  Port=2  SampleTime=SampleTime
  Terminator : Terminator
  Tsamp : SampleTimeMath  TsampMathOp=*  weightValue=0.5  SaturateOnIntegerOverflow=on
  Out1 : Outport  SampleTime=SampleTime
  wires:
  Tsamp/1 -> Out1/1
  Ts/1 -> Terminator/1
  N/1 -> Tsamp/1

== system PIDforVerilog/Discrete PID Controller/Filter/Disc. Trapezoidal Filter Only/Tsamp/External Ts ==
  N : Inport  SampleTime=SampleTime
  Ts : Inport  Port=2  SampleTime=SampleTime
  Gain : Gain  Gain=0.5
  N*Ts Prod Out : Product  OutMin=NTsProdOutMin  OutMax=NTsProdOutMax  SampleTime=SampleTime
  Out1 : Outport  SampleTime=SampleTime
  wires:
  N/1 -> N*Ts Prod Out/1
  N*Ts Prod Out/1 -> Out1/1
  Ts/1 -> Gain/1
  Gain/1 -> N*Ts Prod Out/2

== system PIDforVerilog/Discrete PID Controller/Filter/Disc. Trapezoidal Filter Only/Tsamp/Internal Ts ==
  N : Inport  SampleTime=SampleTime
  Ts : Inport  Port=2  SampleTime=SampleTime
  Terminator : Terminator
  Tsamp : SampleTimeMath  TsampMathOp=*  weightValue=0.5
  Out1 : Outport  SampleTime=SampleTime
  wires:
  N/1 -> Tsamp/1
  Ts/1 -> Terminator/1
  Tsamp/1 -> Out1/1
